simulink model "current_position_feedback"  (R2023b)
settings: Solver=VariableStepAuto  StartTime=0.0  StopTime=2  RelTol=1e-3
libraries: cstblocks x6
settings Model: Creator=frenci  LastModifiedBy=frenci

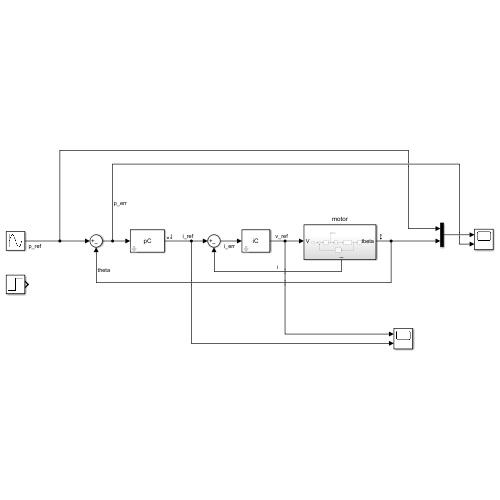
[thumbnail: Simulink's stored preview of the top-level diagram]
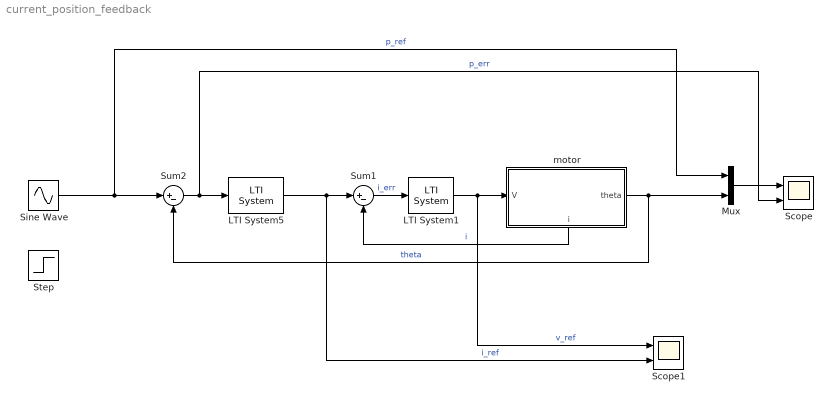
== system current_position_feedback ==
  LTI System1 : cstblocks/LTI System  sys=iC  IC=[]  PadeOrder=0
  LTI System5 : cstblocks/LTI System  sys=pC  IC=[]  PadeOrder=0
  Mux : Mux  Inputs=2
  Scope : Scope  NumInputPorts=2
  Scope1 : Scope  NumInputPorts=2
  Sine Wave : Sin  Frequency=2*pi*100  SampleTime=0
  Step : Step  Time=0.1  SampleTime=0
  Sum1 : Sum  Inputs=|+-
  Sum2 : Sum  Inputs=|+-
  motor : Subsystem
      settings: PortSchema="{\"entries\":[{\"content\":{\"sides\":[{\"content\":{\"connectorIds\":[\"In1\"]},\"type\":\"ConnectorPlacement.EquallySpacedRectSide\",\"uuid\":\"f8a2075c-835e-4141-b12e-4d20e284e554\"},{\"content\":{\"connectorIds\":[\"Out1\"],\"side\":\"RIGHT\"},\"type\":\"ConnectorPlacement.EquallySpacedRectSide\",\"uuid\":\"7d0ccdb0-5eec-43bf-a9a0-3828bb795771\"},{\"content\":{\"side\":\"TOP\"},\"type\":\"ConnectorPlacement.EquallySpacedRectSide\",\"uuid\":\"6f2e9e0d-bcbc-45fe-ae47-d363e6343883\"},{\"content\":{\"connectorIds\":[\"Out2\"],\"side\":\"BOTTOM\"},\"type\":\"ConnectorPlacement.EquallySpacedRectSide\",\"uuid\":\"12f63cf8-6157-4e53-9068-17bec2e9afdd\"}]},\"type\":\"ConnectorPlacement.EquallySpacedConnector\",\"uuid\":\"d79290fb-8e13-45e0-9c36-c4b7a16caadb\"}],\"packageUris\":[\"http://schema.mathworks.com/mf0/Connector/R2020b\"],\"version\":\"1.0\"}"
  wires:
  Sum1/1 -> LTI System1/1  "i_err"
  LTI System5/1 -> Sum1/1, Scope1/2  "i_ref"
  Sum2/1 -> LTI System5/1, Scope/2  "p_err"
  Sine Wave/1 -> Mux/1, Sum2/1  "p_ref"
  Mux/1 -> Scope/1
  motor/1(theta) -> Mux/2, Sum2/2  "theta"
  motor/2(i) -> Sum1/2  "i"
  LTI System1/1 -> Scope1/1, motor/1(V)  "v_ref"

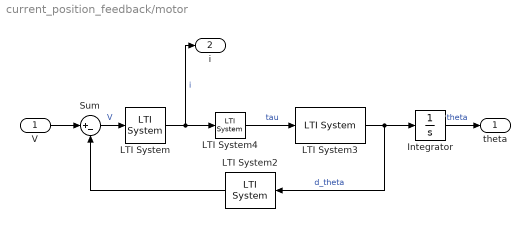
== system current_position_feedback/motor ==
  V : Inport
  Integrator : Integrator
  LTI System : cstblocks/LTI System  sys=El  IC=[]  PadeOrder=0
  LTI System2 : cstblocks/LTI System  sys=Kt  IC=[]  PadeOrder=0
  LTI System3 : cstblocks/LTI System  sys=Me  IC=[]  PadeOrder=0
  LTI System4 : cstblocks/LTI System  sys=Kt  IC=[]  PadeOrder=0
  Sum : Sum  Inputs=|+-
  theta : Outport
  i : Outport  Port=2
  wires:
  LTI System2/1 -> Sum/2
  LTI System4/1 -> LTI System3/1  "tau"
  Integrator/1 -> theta/1  "theta"
  V/1 -> Sum/1
  Sum/1 -> LTI System/1  "V"
  LTI System3/1 -> LTI System2/1, Integrator/1  "d_theta"
  LTI System/1 -> LTI System4/1, i/1  "i"
